simulink model "mech_motorcycle_stability"  (Simulink 6.0)
settings: Solver=ode45  StartTime=0.0  StopTime=3  RelTol=1e-3  AbsTol=1e-6
PreLoadFcn:
  | vu=53;mech_motorcycle_data
values from neighbouring files (symbols this model uses):
  Cf1 = -13.25+1.302*Zf-(1.39e-4)*Zf^2    [mech_motorcycle_data.m]
  Cf2 = 2.788+0.0165*Zf+(3.9e-6)*Zf^2    [mech_motorcycle_data.m]
  Cf3 = -0.06*Zf    [mech_motorcycle_data.m]
  Cfvf = -300+28.577*Zf-0.0143*Zf^2+(1.431e-6)*Zf^3+(3.347e-10)*Zf^4    [mech_motorcycle_data.m]
  Cfvr = -92.9+23.129*Zr-(4.663/1000)*Zr^2-(6.457e-7)*Zr^3+(1.887e-10)*Zr^4    [mech_motorcycle_data.m]
  Cmvf = -0.281+0.2442*Zf+(8.575e-5)*Zf^2    [mech_motorcycle_data.m]
  Cmvr = 9+0.3573*Zr + (3.378e-5)*Zr^2    [mech_motorcycle_data.m]
  Cr1 = 27.38+0.9727*Zr-(4e-6)*Zr^2    [mech_motorcycle_data.m]
  Cr2 = 2.056+0.01282*Zr+(4.928e-6)*Zr^2    [mech_motorcycle_data.m]
  Cr3 = -0.07*Zr    [mech_motorcycle_data.m]
  G = 9.81    [mech_motorcycle_data.m]
  m = 161    [mech_transmission_data.mat]
  Mfw = 26.5    [mech_motorcycle_data.m]    (also in mech_motorcycle_data_nonlinear.m = 25.6)
  Mp = 0.1    [mech_transmission_data.mat]
  Mrw = 26.5    [mech_motorcycle_data.m]    (also in mech_motorcycle_data_nonlinear.m = 25.6)
  N = 270    [mech_transmission_data.mat]
  Rf = 0.336    [mech_motorcycle_data.m]
  Rr = 0.321    [mech_motorcycle_data.m]
  sigmaf = 0.1012+(1.297e-4)*Zf-(3.267e-8)*Zf^2    [mech_motorcycle_data.m]
  sigmar = 0.03594+(1.941e-4)*Zr-(5.667e-8)*Zr^2+(5.728e-12)*Zr^3    [mech_motorcycle_data.m]
  Zf = ((Mf.value*(bb+kk)+Mr.value*bb+Mb.value*(bb-bb_b)+Mp.value*(bb-bb_p))*G-(vu^2)*(Dc.value*hh_cp+Lc.value*whl_bs/2))/whl_bs    [mech_motorcycle_data.m]
  Zr = (Mf.value+Mr.value+Mp.value+Mb.value)*G-Lc.value*vu^2-Zf    [mech_motorcycle_data.m]
undefined symbols (not defined in the file or in its folder): Crr1, Crr2, D_gamma, D_lamda, D_steer, D_v, D_zita, Dc, ifwy, Ifx, Ifxz, Ifz, Ipx, Ipxz, Ipz, irwx, irwy, Irx, Irxz, iry, Irz, k_gamma, k_lamda, k_steer, k_v, k_zita, Lc, Mb, Mf, Mr, rad, s
libraries: mblibv1 x43, simulink x8, aerospace x2
(part 1 of 2)
settings Model: Creator=gwood  LastModifiedBy=batserve  ExtModeAutoUpdateStatusClock=off
settings DataIOCC: SaveState=on  SignalLoggingName=logsOut  OutputTimes=0:0.5:20
settings OptimizationCC: BooleanDataType=off
settings DebuggingCC: CheckExecutionContextPreStartOutputMsg=on  CheckExecutionContextRuntimeOutputMsg=on  SolverPrmCheckMsg=none
settings HardwareCC: TargetUnknown=on

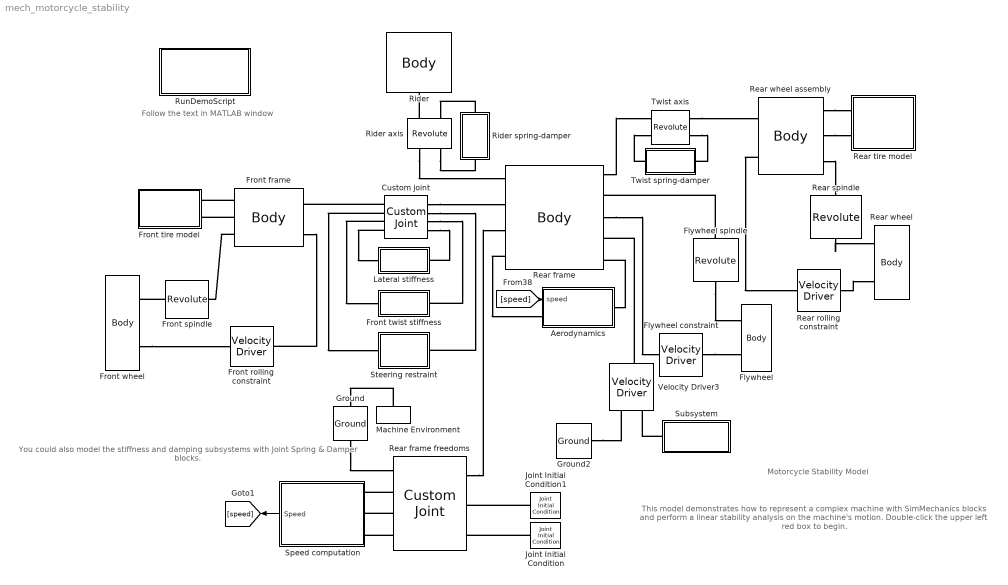
== system mech_motorcycle_stability ==
  note: Motorcycle Stability Model
  note: Follow the text in MATLAB window
  note: This model demonstrates how to represent
      | a complex machine with SimMechanics
      | blocks and perform a linear stability analysis
      | on the machine's motion. Double-click the
      | upper left red box to begin.
  note: You could also model the stiffness
      | and damping subsystems with
      | Joint Spring & Damper blocks.
  Aerodynamics : Subsystem
  Custom joint : mblibv1/Joints/Custom Joint  Orientation=left  PhysicalDomain=mechanical  SubClassName=custom_joint  LeftPortType=blob  RightPortType=blob  LConnTagsString=__newl0|SA1|SA2|SA3  RConnTagsString=__newr0|SA1|SA2|SA3  NumSAPorts=6  CutJoint=off  MarkAsCut=off  Primitives=prismatic_revolute_revolute  PrimitiveProps="P1$WORLD$[0 1 0]$prismatic#R1$WORLD$[cos(epsilon) 0  -sin(epsilon)]$revolute#R2$WORLD$[sin(epsilon) 0 cos(epsilon)]$revolute"  DialogClass=JointBlock
  Flywheel : mblibv1/Bodies/Body  PhysicalDomain=mechanical  SubClassName=Unknown  LeftPortType=workingframe  RightPortType=workingframe  LConnTagsString=CS2|CG  DialogClass=MechanicalBodyBlock  Mass=0  MassUnits=kg  InertiaUnits=kg*m^2  Inertia=[0 0 0;0 iry.value 0;0 0 0]  Shape=Cylinder  ShapeDims=[1 1]  ShapeUnits=m  ShapeUse=false  Density=1  DensityUnits=kg/m^3  DensityUse=false  CG=Left$CG$p1.coordinates$WORLD$WORLD$m$[0 0 0]$Euler X-Y-Z$deg$WORLD$true  WorkingFrames=Left$CS2$p1.coordinates$WORLD$WORLD$m$[0 0 0]$Euler X-Y-Z$deg$WORLD$true
  Flywheel constraint : mblibv1/Constraints &  Drivers/Velocity Driver  PhysicalDomain=mechanical  SubClassName=Unknown  LeftPortType=blob  RightPortType=blob  LConnTagsString=__newl0  RConnTagsString=__newr0  DialogClass=ConstantVelocityConstraint  NumSAPorts=0  Unit_V=m/s  Unit_Omega=rad/s  Coef_V_Base=[1 0 0]  Csys_V_Base=Base  Coef_Omega_Base=[0 0 0]  Csys_Omega_Base=Base  Coef_V_Follower=[0 0 0]  Csys_V_Follower=Follower  Coef_Omega_Follower=Rr*[0 -1 0]  Csys_Omega_Follower=Follower
  Flywheel spindle : mblibv1/Joints/Revolute  Orientation=down  PhysicalDomain=mechanical  SubClassName=Unknown  LeftPortType=blob  RightPortType=blob  LConnTagsString=__newl0  RConnTagsString=__newr0  NumSAPorts=0  CutJoint=off  MarkAsCut=off  Primitives=revolute  PrimitiveProps=R1$WORLD$[0 1 0]$revolute  DialogClass=JointBlock
  Front frame : mblibv1/Bodies/Body  Orientation=left  PhysicalDomain=mechanical  SubClassName=Unknown  LeftPortType=workingframe  RightPortType=workingframe  LConnTagsString=CS1|CS6  RConnTagsString=CS2|CS5|CS3  DialogClass=MechanicalBodyBlock  Mass=Mf.value  MassUnits=kg  InertiaUnits=kg*m^2  Inertia=[Ifx.value 0 Ifxz.value;0 0 0;Ifxz.value 0 Ifz.value]  Shape=Cylinder  ShapeDims=[1 1]  ShapeUnits=m  ShapeUse=false  Density=1  DensityUnits=kg/m^3  DensityUse=false  CG=Left$CG$p3.coordinates$WORLD$WORLD$m$[0 epsilon 0]$Euler X-Y-Z$rad$WORLD$false  WorkingFrames=Left$CS1$p8.coordinates$WORLD$WORLD$m$[0 0 0]$Euler X-Y-Z$deg$WORLD$true#Right$CS2$p11.coordinates$WORLD$WORLD$m$[0 0 0]$Euler X-Y-Z$deg$WORLD$true#Right$CS5$p11.coordinates$WORLD$WORLD$m$[0 0 0]$Euler X-Y-Z$deg$WORLD$true#Right$CS3$p6.coordinates$WORLD$WORLD$m$[0 0 0]$Euler X-Y-Z$deg$WORLD$true#Left$CS6$p6.coordinates$WORLD$WORLD$m$[0 0 0]$Euler X-Y-Z$deg$WORLD$true
  Front rolling constraint : mblibv1/Constraints &  Drivers/Velocity Driver  Orientation=left  PhysicalDomain=mechanical  SubClassName=Unknown  LeftPortType=blob  RightPortType=blob  LConnTagsString=__newl0  RConnTagsString=__newr0  DialogClass=ConstantVelocityConstraint  NumSAPorts=0  Unit_V=m/s  Unit_Omega=rad/s  Coef_V_Base=[1 0 0]  Csys_V_Base=Base  Coef_Omega_Base=[0 0 0]  Csys_Omega_Base=Base  Coef_V_Follower=[0 0 0]  Csys_V_Follower=Follower  Coef_Omega_Follower=Rf*[0 -1 0]  Csys_Omega_Follower=Follower
  Front spindle : mblibv1/Joints/Revolute  Orientation=left  PhysicalDomain=mechanical  SubClassName=Unknown  LeftPortType=blob  RightPortType=blob  LConnTagsString=__newl0  RConnTagsString=__newr0  NumSAPorts=0  CutJoint=off  MarkAsCut=off  Primitives=revolute  PrimitiveProps=R1$WORLD$[0 1 0]$revolute  DialogClass=JointBlock
  Front tire model : Subsystem  Orientation=left
  Front twist stiffness : Subsystem
  Front wheel : mblibv1/Bodies/Body  Orientation=left  PhysicalDomain=mechanical  SubClassName=Unknown  LeftPortType=workingframe  RightPortType=workingframe  LConnTagsString=CS1|CG  DialogClass=MechanicalBodyBlock  Mass=Mfw  MassUnits=kg  InertiaUnits=kg*m^2  Inertia=[0 0 0;0 ifwy.value 0;0 0 0]  Shape=Cylinder  ShapeDims=[1 1]  ShapeUnits=m  ShapeUse=false  Density=1  DensityUnits=kg/m^3  DensityUse=false  CG=Left$CG$p6.coordinates$WORLD$WORLD$m$[0 0 0]$Euler X-Y-Z$deg$WORLD$true  WorkingFrames=Left$CS1$p6.coordinates$WORLD$WORLD$m$[0 0 0]$Euler X-Y-Z$deg$WORLD$true
  Ground : mblibv1/Bodies/Ground  Orientation=down  Opaque=on  LeftPortType=env  RightPortType=workingframe  PhysicalDomain=Mechanical  DialogClass=GroundBlock  CoordPosition=p1.coordinates  CoordPositionUnits=m  StateVectorMgrId=-1  MachineId=[0 0]  ShowEnvPort=on
  Ground2 : mblibv1/Bodies/Ground  Opaque=on  LeftPortType=env  RightPortType=workingframe  PhysicalDomain=Mechanical  DialogClass=GroundBlock  CoordPosition=p7.coordinates  CoordPositionUnits=m  StateVectorMgrId=-1  MachineId=[0 0]  ShowEnvPort=off
  Joint Initial Condition : mblibv1/Sensors &  Actuators/Joint Initial Condition  Orientation=left  Opaque=on  PhysicalDomain=Mechanical  DialogClass=InitialConditionBlock  Primitive=R2  CoordPosition=0.005  Velocity=0.0  AngleUnits=rad  ArcVelocityUnits=rad/s  CoordPositionUnits=m  VelocityUnits=m/s  InitialConditions=P1$false$0$m$rad$0$m/s$rad/s#P2$false$0$m$rad$0$m/s$rad/s#P3$false$0$m$rad$0$m/s$rad/s#R1$false$0$m$rad$0$m/s$rad/s#R2$true$0.005$m$rad$0.0$m/s$rad/s#R3$false$0$m$rad$0$m/s$rad/s#S$false$0$m$rad$0$m/s$rad/s
  Joint Initial Condition1 : mblibv1/Sensors &  Actuators/Joint Initial Condition  Orientation=left  Opaque=on  PhysicalDomain=Mechanical  DialogClass=InitialConditionBlock  Primitive=R1  CoordPosition=0.0  Velocity=0.0  AngleUnits=rad  ArcVelocityUnits=rad/s  CoordPositionUnits=m  VelocityUnits=m/s  InitialConditions=P1$false$0$m$rad$0$m/s$rad/s#P2$false$0$m$rad$0$m/s$rad/s#P3$false$0$m$rad$0$m/s$rad/s#R1$true$0.0$m$rad$0.0$m/s$rad/s#R2$false$0$m$rad$0$m/s$rad/s#R3$false$0$m$rad$0$m/s$rad/s#S$false$0$m$rad$0$m/s$rad/s
  Lateral stiffness : Subsystem
  Machine Environment : mblibv1/Bodies/Machine Environment  Tag=Factory ground  Orientation=up  DialogController=MECH.DialogSource  Opaque=on  PortType=env  PhysicalDomain=Mechanical  DialogTemplateClass=MECH.MachineEnvironment  SyncWhenCopied=off  Gravity=[0;0;G]  GravityUnits=m/s^2  GravityAsSignal=off  Dimensionality=3D Only  AnalysisType=Forward dynamics  LinearAssemblyTolerance=1e-3  LinearAssemblyToleranceUnits=m  AngularAssemblyTolerance=1e-3  AngularAssemblyToleranceUnits=rad  ConstraintSolverType=Stabilizing  ConstraintRelTolerance=1e-4  ConstraintAbsTolerance=1e-4  UseRobustSingularityHandling=off  StatePerturbationType=Fixed  PerturbationSize=1e-5  VisualizeMachine=on
  Rear spindle : mblibv1/Joints/Revolute  Orientation=down  PhysicalDomain=mechanical  SubClassName=Unknown  LeftPortType=blob  RightPortType=blob  LConnTagsString=__newl0  RConnTagsString=__newr0  NumSAPorts=0  CutJoint=off  MarkAsCut=off  Primitives=revolute  PrimitiveProps=R1$WORLD$[0 1 0]$revolute  DialogClass=JointBlock
  Rear frame : mblibv1/Bodies/Body  PhysicalDomain=mechanical  SubClassName=Unknown  LeftPortType=workingframe  RightPortType=workingframe  LConnTagsString=CS1|CS3|CS6|CS9  RConnTagsString=CS2|CS7|CS8|CS11|CS10  DialogClass=MechanicalBodyBlock  Mass=Mr.value  MassUnits=kg  InertiaUnits=kg*m^2  Inertia=[Irx.value 0 Irxz.value;0 0 0;Irxz.value 0 Irz.value]  Shape=Cylinder  ShapeDims=[1 1]  ShapeUnits=m  ShapeUse=false  Density=1  DensityUnits=kg/m^3  DensityUse=false  CG=Right$CG$p1.coordinates$WORLD$WORLD$m$[0 0 0]$Euler X-Y-Z$deg$WORLD$false  WorkingFrames=Left$CS1$p9.coordinates$WORLD$WORLD$m$[0 0 0]$Euler X-Y-Z$deg$WORLD$true#Right$CS2$p7.coordinates$WORLD$WORLD$m$[0 0 0]$Euler X-Y-Z$deg$WORLD$true#Left$CS3$p8.coordinates$WORLD$WORLD$m$[0 0 0]$Euler X-Y-Z$deg$WORLD$true#Left$CS6$p1.coordinates$WORLD$WORLD$m$[0 0 0]$Euler X-Y-Z$deg$WORLD$true#Right$CS7$p1.coordinates$WORLD$WORLD$m$[0 0 0]$Euler X-Y-Z$deg$WORLD$true#Right$CS8$p1.coordinates$WORLD$WORLD$m$[0 0 0]$Euler X-Y-Z$deg$WORLD$true#Right$CS11$p10.coordinates$WORLD$WORLD$m$[0 0 0]$Euler X-Y-Z$deg$WORLD$true#Left$CS9$p12.coordinates$WORLD$WORLD$m$[0 0 0]$Euler X-Y-Z$deg$WORLD$true#Right$CS10$p12.coordinates$WORLD$WORLD$m$[0 0 0]$Euler X-Y-Z$deg$WORLD$true
  Rear frame freedoms : mblibv1/Joints/Custom Joint  PhysicalDomain=mechanical  SubClassName=custom_joint  LeftPortType=blob  RightPortType=blob  LConnTagsString=__newl0|SA1|SA2|SA3  RConnTagsString=__newr0|SA1|SA2  NumSAPorts=5  CutJoint=off  MarkAsCut=off  Primitives=prismatic_prismatic_revolute_revolute  PrimitiveProps=P1$WORLD$[1 0 0]$prismatic#P2$WORLD$[0 1 0]$prismatic#R1$WORLD$[0 0 1]$revolute#R2$WORLD$[1 0 0]$revolute  DialogClass=JointBlock
  Rear rolling constraint : mblibv1/Constraints &  Drivers/Velocity Driver  PhysicalDomain=mechanical  SubClassName=Unknown  LeftPortType=blob  RightPortType=blob  LConnTagsString=__newl0  RConnTagsString=__newr0  DialogClass=ConstantVelocityConstraint  NumSAPorts=0  Unit_V=m/s  Unit_Omega=rad/s  Coef_V_Base=[1 0 0]  Csys_V_Base=Base  Coef_Omega_Base=[0 0 0]  Csys_Omega_Base=Base  Coef_V_Follower=[0 0 0]  Csys_V_Follower=Follower  Coef_Omega_Follower=Rr*[0 -1 0]  Csys_Omega_Follower=Follower
  Rear tire model : Subsystem
  Rear wheel : mblibv1/Bodies/Body  PhysicalDomain=mechanical  SubClassName=Unknown  LeftPortType=workingframe  RightPortType=workingframe  LConnTagsString=CS1|CG  DialogClass=MechanicalBodyBlock  Mass=Mrw  MassUnits=kg  InertiaUnits=kg*m^2  Inertia=[irwx.value 0 0;0 irwy.value 0;0 0 irwx.value]  Shape=Cylinder  ShapeDims=[1 1]  ShapeUnits=m  ShapeUse=false  Density=1  DensityUnits=kg/m^3  DensityUse=false  CG=Left$CG$p5.coordinates$WORLD$WORLD$m$[0 0 0]$Euler X-Y-Z$deg$WORLD$true  WorkingFrames=Left$CS1$p5.coordinates$WORLD$WORLD$m$[0 0 0]$Euler X-Y-Z$deg$WORLD$true
  Rear wheel assembly : mblibv1/Bodies/Body  PhysicalDomain=mechanical  SubClassName=Unknown  LeftPortType=workingframe  RightPortType=workingframe  LConnTagsString=CS1|CS6  RConnTagsString=CS2|CS5|CS3  DialogClass=MechanicalBodyBlock  Mass=Mb.value  MassUnits=kg  InertiaUnits=kg*m^2  Inertia=zeros(3,3)  Shape=Cylinder  ShapeDims=[1 1]  ShapeUnits=m  ShapeUse=false  Density=1  DensityUnits=kg/m^3  DensityUse=false  CG=Left$CG$p2.coordinates$WORLD$WORLD$m$[0 0 0]$Euler X-Y-Z$deg$WORLD$false  WorkingFrames=Left$CS1$p7.coordinates$WORLD$WORLD$m$[0 0 0]$Euler X-Y-Z$deg$WORLD$true#Right$CS2$p10.coordinates$WORLD$WORLD$m$[0 0 0]$Euler X-Y-Z$deg$WORLD$true#Right$CS5$p10.coordinates$WORLD$WORLD$m$[0 0 0]$Euler X-Y-Z$deg$WORLD$true#Right$CS3$p5.coordinates$WORLD$WORLD$m$[0 0 0]$Euler X-Y-Z$deg$WORLD$true#Left$CS6$p5.coordinates$WORLD$WORLD$m$[0 0 0]$Euler X-Y-Z$deg$WORLD$true
  Rider : mblibv1/Bodies/Body  Orientation=up  PhysicalDomain=mechanical  SubClassName=Unknown  LeftPortType=workingframe  RightPortType=workingframe  LConnTagsString=CS1  DialogClass=MechanicalBodyBlock  Mass=Mp.value  MassUnits=kg  InertiaUnits=kg*m^2  Inertia=[Ipx.value 0 Ipxz.value;0 0 0;Ipxz.value 0 Ipz.value]  Shape=Cylinder  ShapeDims=[1 1]  ShapeUnits=m  ShapeUse=false  Density=1  DensityUnits=kg/m^3  DensityUse=false  CG=Left$CG$p4.coordinates$WORLD$WORLD$m$[0 0 0]$Euler X-Y-Z$deg$WORLD$false  WorkingFrames=Left$CS1$p9.coordinates$WORLD$WORLD$m$[0 0 0]$Euler X-Y-Z$deg$WORLD$true
  Rider axis : mblibv1/Joints/Revolute  Orientation=up  PhysicalDomain=mechanical  SubClassName=Unknown  LeftPortType=blob  RightPortType=blob  LConnTagsString=__newl0|SA1  RConnTagsString=__newr0|SA1  NumSAPorts=2  CutJoint=off  MarkAsCut=off  Primitives=revolute  PrimitiveProps=R1$WORLD$[1 0 0]$revolute  DialogClass=JointBlock
  Rider spring-damper : Subsystem  Orientation=down
  RunDemoScript : Subsystem
      settings: OpenFcn=mech_motorcycle_stability_demo
      mask Display: disp('Double-click\nhere to\nstart Demo')
  Speed computation : Subsystem  Orientation=left
  Steering restraint : Subsystem
  Subsystem : Subsystem  Orientation=left
  Twist axis : mblibv1/Joints/Revolute  PhysicalDomain=mechanical  SubClassName=Unknown  LeftPortType=blob  RightPortType=blob  LConnTagsString=__newl0|SA1  RConnTagsString=__newr0|SA1  NumSAPorts=2  CutJoint=off  MarkAsCut=off  Primitives=revolute  PrimitiveProps=R1$WORLD$[sin(epsilon1) 0 cos(epsilon1)]$revolute  DialogClass=JointBlock
  Twist spring-damper : Subsystem
  Velocity Driver3 : mblibv1/Constraints &  Drivers/Velocity Driver  Orientation=up  PhysicalDomain=mechanical  SubClassName=Unknown  LeftPortType=blob  RightPortType=blob  LConnTagsString=__newl0|SA1  RConnTagsString=__newr0  DialogClass=ConstantVelocityConstraint  NumSAPorts=1  Unit_V=m/s  Unit_Omega=rad/s  Coef_V_Base=[1 0 0]  Csys_V_Base=Base  Coef_Omega_Base=[0 0 0]  Csys_Omega_Base=Base  Coef_V_Follower=[1 0 0]  Csys_V_Follower=Follower  Coef_Omega_Follower=[0 0 0]  Csys_Omega_Follower=Follower
  wires:
  [speed] -> Aerodynamics/1(speed)
  Speed computation/1(Speed) -> [speed]
  connections:
  Rider axis/LConn1 -- Rear frame/LConn1
  Custom joint/LConn1 -- Rear frame/LConn2
  Front frame/RConn3 -- Front spindle/LConn1
  Custom joint/RConn1 -- Front frame/LConn1
  Rider axis/LConn2 -- Rider spring-damper/RConn1
  Rider axis/RConn1 -- Rider/LConn1
  Rider spring-damper/LConn1 -- Rider axis/RConn2
  Custom joint/LConn4 -- Lateral stiffness/RConn1
  Custom joint/RConn4 -- Lateral stiffness/LConn1
  Custom joint/RConn3 -- Front twist stiffness/LConn1
  Custom joint/LConn3 -- Front twist stiffness/RConn1
  Custom joint/LConn2 -- Steering restraint/RConn1
  Custom joint/RConn2 -- Steering restraint/LConn1
  Front frame/RConn1 -- Front tire model/LConn1
  Front frame/RConn2 -- Front tire model/LConn2
  Rear wheel assembly/RConn3 -- Rear spindle/LConn1
  Twist axis/RConn1 -- Rear wheel assembly/LConn1
  Rear frame/LConn4 -- Aerodynamics/LConn1
  Front frame/LConn2 -- Front rolling constraint/LConn1
  Rear wheel assembly/LConn2 -- Rear rolling constraint/LConn1
  Flywheel spindle/LConn1 -- Rear frame/RConn2
  Rear frame/RConn3 -- Flywheel constraint/LConn1
  Velocity Driver3/RConn1 -- Rear frame/RConn4
  Front spindle/RConn1 -- Front wheel/LConn1
  Front wheel/LConn2 -- Front rolling constraint/RConn1
  Rear frame freedoms/RConn1 -- Rear frame/LConn3
  Ground/RConn1 -- Rear frame freedoms/LConn1
  Rear frame freedoms/LConn2 -- Speed computation/LConn1
  Rear frame freedoms/LConn3 -- Speed computation/LConn2
  Rear frame freedoms/LConn4 -- Speed computation/LConn3
  Joint Initial Condition/RConn1 -- Rear frame freedoms/RConn3
  Joint Initial Condition1/RConn1 -- Rear frame freedoms/RConn2
  Aerodynamics/RConn1 -- Rear frame/RConn5
  Twist axis/RConn2 -- Twist spring-damper/RConn1
  Rear wheel assembly/RConn1 -- Rear tire model/LConn1
  Rear wheel assembly/RConn2 -- Rear tire model/LConn2
  Ground2/RConn1 -- Velocity Driver3/LConn1
  Subsystem/RConn1 -- Velocity Driver3/LConn2
  Rear spindle/RConn1 -- Rear wheel/LConn1
  Rear rolling constraint/RConn1 -- Rear wheel/LConn2
  Flywheel spindle/RConn1 -- Flywheel/LConn1
  Flywheel constraint/RConn1 -- Flywheel/LConn2
  Rear frame/RConn1 -- Twist axis/LConn1
  Twist spring-damper/LConn1 -- Twist axis/LConn2
  Machine Environment/RConn1 -- Ground/LConn1

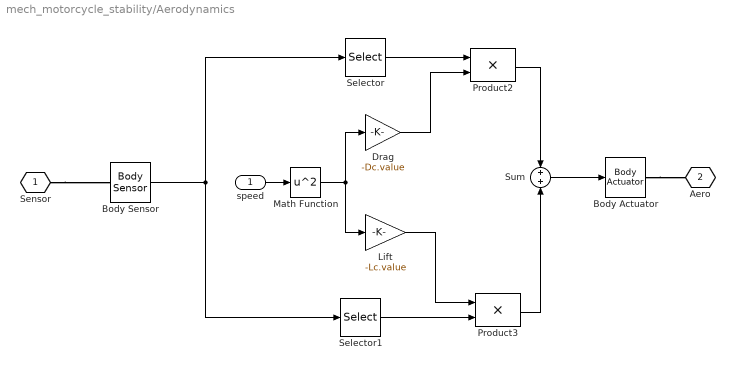
== system mech_motorcycle_stability/Aerodynamics ==
  speed : Inport  Port=1  LatchInput=off
  Body Actuator : mblibv1/Sensors &  Actuators/Body Actuator  Opaque=on  PhysicalDomain=Mechanical  PortType=blob  ActuationStyle=Force  AngleUnits=deg  ArcVelocityUnits=deg/s  ArcAccelerationUnits=deg/s^2  CoordPositionUnits=m  VelocityUnits=m/s  AccelerationUnits=m/s^2  ForceUnits=N  TorqueUnits=N-m  ActiveIO=on  Width=3  DialogClass=MechanicalActuatorBlock  ReferenceFrame=Absolute (World)  Angle=off  CoordPosition=on  Force=on  Torque=off
  Body Sensor : mblibv1/Sensors &  Actuators/Body Sensor  Opaque=on  PhysicalDomain=Mechanical  PortType=blob  Muxed=on  Pose=on  Angle=on  AngleUnits=deg  ArcVelocity=off  ArcVelocityUnits=deg/s  ArcAcceleration=off  ArcAccelerationUnits=deg/s^2  CoordPosition=off  CoordPositionUnits=m  Velocity=off  VelocityUnits=m/s  Acceleration=off  AccelerationUnits=m/s^2  Quaternion=on  QuaternionDT=off  QuaternionDDT=off  QuaternionUnits=off  OutputVector=[ 9 ]  ActiveIO=on  Width=9  DialogClass=MechanicalSensorBlock  ReferenceFrame=Absolute (World)
  Drag : Gain  Gain=-Dc.value  SaturateOnIntegerOverflow=on
  Lift : Gain  Gain=-Lc.value  SaturateOnIntegerOverflow=on
  Math Function : Math  Operator=square  SaturateOnIntegerOverflow=on
  Product2 : Product  SaturateOnIntegerOverflow=on  InputSameDT=on
  Product3 : Product  SaturateOnIntegerOverflow=on  InputSameDT=on
  Selector : Selector  Elements=[1:3]  InputPortWidth=9
  Selector1 : Selector  Elements=[7:9]  InputPortWidth=9
  Sum : Sum  SaturateOnIntegerOverflow=on  InputSameDT=on
  Sensor : PMIOPort  Port=1  Side=Left
  Aero : PMIOPort  Orientation=left  Port=2  Side=Right
  wires:
  speed/1 -> Math Function/1
  Math Function/1 -> Drag/1, Lift/1
  Lift/1 -> Product3/1
  Selector/1 -> Product2/1
  Body Sensor/1 -> Selector/1, Selector1/1
  Sum/1 -> Body Actuator/1
  Product2/1 -> Sum/1
  Product3/1 -> Sum/2
  Drag/1 -> Product2/2
  Selector1/1 -> Product3/2
  connections:
  Body Actuator/RConn1 -- Aero/RConn1
  Sensor/RConn1 -- Body Sensor/LConn1

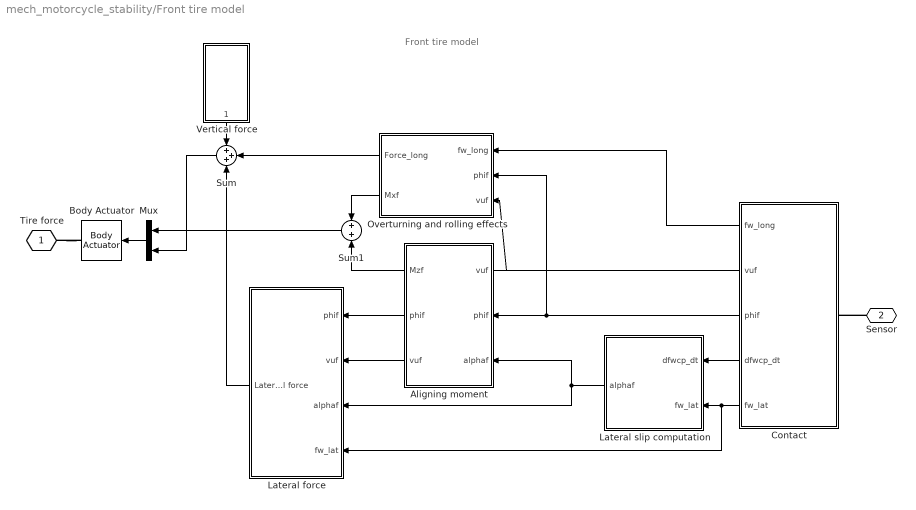
== system mech_motorcycle_stability/Front tire model ==
  note: Front tire model
  Aligning moment : Subsystem  Orientation=left
  Body Actuator : mblibv1/Sensors &  Actuators/Body Actuator  Orientation=left  Opaque=on  PhysicalDomain=Mechanical  PortType=blob  ActuationStyle=Force  AngleUnits=deg  ArcVelocityUnits=deg/s  ArcAccelerationUnits=deg/s^2  CoordPositionUnits=m  VelocityUnits=m/s  AccelerationUnits=m/s^2  ForceUnits=N  TorqueUnits=N-m  ActiveIO=on  Width=6  DialogClass=MechanicalActuatorBlock  ReferenceFrame=Absolute (World)  Angle=off  CoordPosition=off  Force=on  Torque=on
  Contact : Subsystem  Orientation=left
  Lateral force : Subsystem  Orientation=left
  Lateral slip computation : Subsystem  Orientation=left
  Mux : Mux  Orientation=left  Inputs=2
  Overturning and rolling effects : Subsystem  Orientation=left
  Sum : Sum  Orientation=left  Inputs=+++  SaturateOnIntegerOverflow=on  InputSameDT=on
  Sum1 : Sum  Orientation=left  SaturateOnIntegerOverflow=on  InputSameDT=on
  Vertical force : Subsystem  Orientation=down
  Tire force : PMIOPort  Tag=PMCPort  Port=1  Side=Left
  Sensor : PMIOPort  Orientation=left  Port=2  Side=Left
  wires:
  Vertical force/1(Force_vert) -> Sum/1
  Aligning moment/3("vuf ") -> Lateral force/2(vuf)
  Aligning moment/2("phif ") -> Lateral force/1(phif)
  Aligning moment/1(Mzf) -> Sum1/2
  Overturning and rolling effects/2(Mxf) -> Sum1/1
  Lateral force/1(Lateral force) -> Sum/3
  Overturning and rolling effects/1(Force_long) -> Sum/2
  Contact/4(dfwcp_dt) -> Lateral slip computation/1(dfwcp_dt)
  Contact/5(fw_lat) -> Lateral slip computation/2(fw_lat), Lateral force/4(fw_lat)
  Contact/3(phif) -> Aligning moment/2(phif), Overturning and rolling effects/2(phif)
  Contact/1(fw_long) -> Overturning and rolling effects/1(fw_long)
  Contact/2(vuf) -> Aligning moment/1(vuf), Overturning and rolling effects/3(vuf)
  Lateral slip computation/1(alphaf) -> Aligning moment/3(alphaf), Lateral force/3(alphaf)
  Sum1/1 -> Mux/1
  Sum/1 -> Mux/2
  Mux/1 -> Body Actuator/1
  connections:
  Body Actuator/RConn1 -- Tire force/RConn1
  Sensor/RConn1 -- Contact/LConn1

== system mech_motorcycle_stability/Front twist stiffness ==
  note: Twist stiffness model for bending flexibility
  note: Press any key to continue
  Damping : Gain  Gain=-D_gamma.value  SaturateOnIntegerOverflow=on
  Demux : Demux  Outputs=2
  Initial Force : Constant  Value=0
  Joint Actuator : mblibv1/Sensors &  Actuators/Joint Actuator  Opaque=on  PhysicalDomain=Mechanical  PortType=blob  ActuationStyle=Force  AngleUnits=rad  ArcVelocityUnits=rad/s  ArcAccelerationUnits=rad/s^2  CoordPositionUnits=m  VelocityUnits=m/s  AccelerationUnits=m/s^2  ForceUnits=N  TorqueUnits=N-m  ActiveIO=on  Width=1  DialogClass=MechanicalActuatorBlock  Primitive=R1  ReferenceFrame=Absolute (INERTIAL)
  Joint Sensor : mblibv1/Sensors &  Actuators/Joint Sensor  Opaque=on  PhysicalDomain=Mechanical  PortType=blob  Muxed=on  Pose=off  Angle=on  AngleUnits=rad  ArcVelocity=on  ArcVelocityUnits=rad/s  ArcAcceleration=off  ArcAccelerationUnits=deg/s^2  CoordPosition=on  CoordPositionUnits=m  Velocity=on  VelocityUnits=m/s  Acceleration=off  AccelerationUnits=m/s^2  Quaternion=on  QuaternionDT=off  QuaternionDDT=off  QuaternionUnits=off  OutputVector=[ 1 1 ]  ActiveIO=on  Width=2  DialogClass=MechanicalSensorBlock  Primitive=R1  Force=off  ForceUnits=N  Torque=off  TorqueUnits=N-m  ReferenceFrame=Absolute (INERTIAL)  ReactionSensedSide=Base  ReactionReferenceFrame=Absolute (World)  ReactionForce=off  ReactionForceUnits=N  ReactionMoment=off  ReactionMomentUnits=N-m
  Stiffness : Gain  Gain=-k_gamma.value  SaturateOnIntegerOverflow=on
  Sum : Sum  Inputs=+++  SaturateOnIntegerOverflow=on  InputSameDT=on
  S : PMIOPort  Port=1  Side=Left
  A : PMIOPort  Orientation=left  Port=2  Side=Right
  wires:
  Joint Sensor/1 -> Demux/1
  Demux/1 -> Stiffness/1  "Rotation (rad)"
  Demux/2 -> Damping/1  "Rotation rate (rad/s)"
  Damping/1 -> Sum/2
  Stiffness/1 -> Sum/1
  Initial Force/1 -> Sum/3
  Sum/1 -> Joint Actuator/1  "Torque (Nm)"
  connections:
  S/RConn1 -- Joint Sensor/LConn1
  Joint Actuator/RConn1 -- A/RConn1

== system mech_motorcycle_stability/Lateral stiffness ==
  note: Lateral stiffness model for transverse flexibility
  note: Press any key to continue
  Damping : Gain  Gain=-D_v.value  SaturateOnIntegerOverflow=on
  Demux : Demux  Outputs=2
  Initial Force : Constant  Value=0
  Joint Actuator : mblibv1/Sensors &  Actuators/Joint Actuator  Opaque=on  PhysicalDomain=Mechanical  PortType=blob  ActuationStyle=Force  AngleUnits=rad  ArcVelocityUnits=rad/s  ArcAccelerationUnits=rad/s^2  CoordPositionUnits=m  VelocityUnits=m/s  AccelerationUnits=m/s^2  ForceUnits=N  TorqueUnits=N-m  ActiveIO=on  Width=1  DialogClass=MechanicalActuatorBlock  Primitive=P1  ReferenceFrame=Absolute (INERTIAL)
  Joint Sensor : mblibv1/Sensors &  Actuators/Joint Sensor  Opaque=on  PhysicalDomain=Mechanical  PortType=blob  Muxed=on  Pose=off  Angle=on  AngleUnits=rad  ArcVelocity=on  ArcVelocityUnits=rad/s  ArcAcceleration=off  ArcAccelerationUnits=deg/s^2  CoordPosition=on  CoordPositionUnits=m  Velocity=on  VelocityUnits=m/s  Acceleration=off  AccelerationUnits=m/s^2  Quaternion=on  QuaternionDT=off  QuaternionDDT=off  QuaternionUnits=off  OutputVector=[ 1 1 ]  ActiveIO=on  Width=2  DialogClass=MechanicalSensorBlock  Primitive=P1  Force=off  ForceUnits=N  Torque=off  TorqueUnits=N-m  ReferenceFrame=Absolute (INERTIAL)  ReactionSensedSide=Base  ReactionReferenceFrame=Absolute (World)  ReactionForce=off  ReactionForceUnits=N  ReactionMoment=off  ReactionMomentUnits=N-m
  Stiffness : Gain  Gain=-k_v.value  SaturateOnIntegerOverflow=on
  Sum : Sum  Inputs=+++  SaturateOnIntegerOverflow=on  InputSameDT=on
  S : PMIOPort  Port=1  Side=Left
  A : PMIOPort  Orientation=left  Port=2  Side=Right
  wires:
  Initial Force/1 -> Sum/3
  Stiffness/1 -> Sum/1
  Damping/1 -> Sum/2
  Demux/2 -> Damping/1  "Velocity (m/s)"
  Demux/1 -> Stiffness/1  "Displacement (m)"
  Joint Sensor/1 -> Demux/1
  Sum/1 -> Joint Actuator/1  "Lateral force (N)"
  connections:
  Joint Actuator/RConn1 -- A/RConn1
  S/RConn1 -- Joint Sensor/LConn1

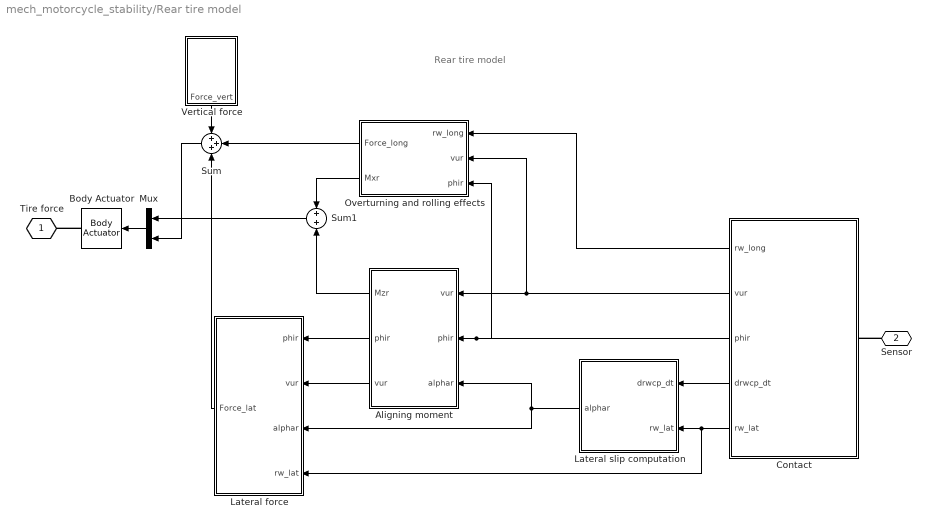
== system mech_motorcycle_stability/Rear tire model ==
  note: Rear tire model
  Aligning moment : Subsystem  Orientation=left
  Body Actuator : mblibv1/Sensors &  Actuators/Body Actuator  Orientation=left  Opaque=on  PhysicalDomain=Mechanical  PortType=blob  ActuationStyle=Force  AngleUnits=deg  ArcVelocityUnits=deg/s  ArcAccelerationUnits=deg/s^2  CoordPositionUnits=m  VelocityUnits=m/s  AccelerationUnits=m/s^2  ForceUnits=N  TorqueUnits=N-m  ActiveIO=on  Width=6  DialogClass=MechanicalActuatorBlock  ReferenceFrame=Absolute (World)  Angle=off  CoordPosition=off  Force=on  Torque=on
  Contact : Subsystem  Orientation=left
  Lateral force : Subsystem  Orientation=left
  Lateral slip computation : Subsystem  Orientation=left
  Mux : Mux  Orientation=left  Inputs=2
  Overturning and rolling effects : Subsystem  Orientation=left
  Sum : Sum  Orientation=left  Inputs=+++  SaturateOnIntegerOverflow=on  InputSameDT=on
  Sum1 : Sum  Orientation=left  SaturateOnIntegerOverflow=on  InputSameDT=on
  Vertical force : Subsystem  Orientation=down
  Tire force : PMIOPort  Tag=PMCPort  Port=1  Side=Left
  Sensor : PMIOPort  Orientation=left  Port=2  Side=Left
  wires:
  Aligning moment/2("phir ") -> Lateral force/1(phir)
  Aligning moment/3("vur ") -> Lateral force/2(vur)
  Aligning moment/1(Mzr) -> Sum1/2
  Overturning and rolling effects/2(Mxr) -> Sum1/1
  Lateral force/1(Force_lat) -> Sum/3
  Overturning and rolling effects/1(Force_long) -> Sum/2
  Contact/4(drwcp_dt) -> Lateral slip computation/1(drwcp_dt)
  Contact/5(rw_lat) -> Lateral slip computation/2(rw_lat), Lateral force/4(rw_lat)
  Contact/3(phir) -> Aligning moment/2(phir), Overturning and rolling effects/3(phir)
  Contact/2(vur) -> Aligning moment/1(vur), Overturning and rolling effects/2(vur)
  Contact/1(rw_long) -> Overturning and rolling effects/1(rw_long)
  Sum1/1 -> Mux/1
  Sum/1 -> Mux/2
  Mux/1 -> Body Actuator/1
  Vertical force/1(Force_vert) -> Sum/1
  Lateral slip computation/1(alphar) -> Aligning moment/3(alphar), Lateral force/3(alphar)
  connections:
  Sensor/RConn1 -- Contact/LConn1
  Body Actuator/RConn1 -- Tire force/RConn1

== system mech_motorcycle_stability/Rider spring-damper ==
  note: Rider stiffness and damping model
  note: Press any key to continue
  Damping : Gain  Gain=-D_zita.value  SaturateOnIntegerOverflow=on
  Demux : Demux  Outputs=2
  Initial Force : Constant  Value=0
  Joint Actuator : mblibv1/Sensors &  Actuators/Joint Actuator  Opaque=on  PhysicalDomain=Mechanical  PortType=blob  ActuationStyle=Force  AngleUnits=deg  ArcVelocityUnits=deg/s  ArcAccelerationUnits=deg/s^2  CoordPositionUnits=m  VelocityUnits=m/s  AccelerationUnits=m/s^2  ForceUnits=N  TorqueUnits=N-m  ActiveIO=on  Width=1  DialogClass=MechanicalActuatorBlock  Primitive=R1  ReferenceFrame=Absolute (INERTIAL)
  Joint Sensor : mblibv1/Sensors &  Actuators/Joint Sensor  Opaque=on  PhysicalDomain=Mechanical  PortType=blob  Muxed=on  Pose=off  Angle=on  AngleUnits=rad  ArcVelocity=on  ArcVelocityUnits=rad/s  ArcAcceleration=off  ArcAccelerationUnits=deg/s^2  CoordPosition=on  CoordPositionUnits=m  Velocity=on  VelocityUnits=m/s  Acceleration=off  AccelerationUnits=m/s^2  Quaternion=on  QuaternionDT=off  QuaternionDDT=off  QuaternionUnits=off  OutputVector=[ 1 1 ]  ActiveIO=on  Width=2  DialogClass=MechanicalSensorBlock  Primitive=R1  Force=off  ForceUnits=N  Torque=off  TorqueUnits=N-m  ReferenceFrame=Absolute (INERTIAL)  ReactionSensedSide=Base  ReactionReferenceFrame=Absolute (World)  ReactionForce=off  ReactionForceUnits=N  ReactionMoment=off  ReactionMomentUnits=N-m
  Stiffness : Gain  Gain=-k_zita.value  SaturateOnIntegerOverflow=on
  Sum : Sum  Inputs=+++  SaturateOnIntegerOverflow=on  InputSameDT=on
  S : PMIOPort  Port=1  Side=Left
  A : PMIOPort  Orientation=left  Port=2  Side=Right
  wires:
  Sum/1 -> Joint Actuator/1  "Torque (Nm)"
  Initial Force/1 -> Sum/3
  Stiffness/1 -> Sum/1
  Damping/1 -> Sum/2
  Demux/2 -> Damping/1  "Angular velocity (rad/s)"
  Demux/1 -> Stiffness/1  "Angle (rad)"
  Joint Sensor/1 -> Demux/1
  connections:
  Joint Actuator/RConn1 -- A/RConn1
  S/RConn1 -- Joint Sensor/LConn1

== system mech_motorcycle_stability/RunDemoScript ==

== system mech_motorcycle_stability/Speed computation ==
  Joint Sensor : mblibv1/Sensors &  Actuators/Joint Sensor  Orientation=left  Opaque=on  PhysicalDomain=Mechanical  PortType=blob  Muxed=on  Pose=off  Angle=on  AngleUnits=deg  ArcVelocity=off  ArcVelocityUnits=deg/s  ArcAcceleration=off  ArcAccelerationUnits=deg/s^2  CoordPosition=off  CoordPositionUnits=m  Velocity=on  VelocityUnits=m/s  Acceleration=off  AccelerationUnits=m/s^2  Quaternion=on  QuaternionDT=off  QuaternionDDT=off  QuaternionUnits=off  OutputVector=[ 1 ]  ActiveIO=on  Width=1  DialogClass=MechanicalSensorBlock  Primitive=P1  Force=off  ForceUnits=N  Torque=off  TorqueUnits=N-m  ReferenceFrame=Absolute (INERTIAL)  ReactionSensedSide=Base  ReactionReferenceFrame=Absolute (World)  ReactionForce=off  ReactionForceUnits=N  ReactionMoment=off  ReactionMomentUnits=N-m
  Joint Sensor1 : mblibv1/Sensors &  Actuators/Joint Sensor  Orientation=left  Opaque=on  PhysicalDomain=Mechanical  PortType=blob  Muxed=on  Pose=off  Angle=on  AngleUnits=deg  ArcVelocity=off  ArcVelocityUnits=deg/s  ArcAcceleration=off  ArcAccelerationUnits=deg/s^2  CoordPosition=off  CoordPositionUnits=m  Velocity=on  VelocityUnits=m/s  Acceleration=off  AccelerationUnits=m/s^2  Quaternion=on  QuaternionDT=off  QuaternionDDT=off  QuaternionUnits=off  OutputVector=[ 1 ]  ActiveIO=on  Width=1  DialogClass=MechanicalSensorBlock  Primitive=P2  Force=off  ForceUnits=N  Torque=off  TorqueUnits=N-m  ReferenceFrame=Absolute (INERTIAL)  ReactionSensedSide=Base  ReactionReferenceFrame=Absolute (World)  ReactionForce=off  ReactionForceUnits=N  ReactionMoment=off  ReactionMomentUnits=N-m
  Joint Sensor2 : mblibv1/Sensors &  Actuators/Joint Sensor  Orientation=left  Opaque=on  PhysicalDomain=Mechanical  PortType=blob  Muxed=on  Pose=off  Angle=on  AngleUnits=rad  ArcVelocity=off  ArcVelocityUnits=rad/s  ArcAcceleration=off  ArcAccelerationUnits=deg/s^2  CoordPosition=off  CoordPositionUnits=m  Velocity=on  VelocityUnits=m/s  Acceleration=off  AccelerationUnits=m/s^2  Quaternion=on  QuaternionDT=off  QuaternionDDT=off  QuaternionUnits=off  OutputVector=[ 1 ]  ActiveIO=on  Width=1  DialogClass=MechanicalSensorBlock  Primitive=R1  Force=off  ForceUnits=N  Torque=off  TorqueUnits=N-m  ReferenceFrame=Absolute (INERTIAL)  ReactionSensedSide=Base  ReactionReferenceFrame=Absolute (World)  ReactionForce=off  ReactionForceUnits=N  ReactionMoment=off  ReactionMomentUnits=N-m
  Product : Product  Orientation=left  SaturateOnIntegerOverflow=on  InputSameDT=on
  Product1 : Product  Orientation=left  SaturateOnIntegerOverflow=on  InputSameDT=on
  Sum : Sum  Orientation=left  Inputs=|++  SaturateOnIntegerOverflow=on  InputSameDT=on
  Trigonometric Function : Trigonometry  Orientation=left  Operator=cos
  Trigonometric Function1 : Trigonometry  Orientation=left
  Sensor1 : PMIOPort  Orientation=left  Port=1  Side=Left
  Sensor2 : PMIOPort  Orientation=left  Port=2  Side=Left
  Sensor3 : PMIOPort  Orientation=left  Port=3  Side=Left
  Speed : Outport  Orientation=left
  wires:
  Joint Sensor/1 -> Product/1
  Joint Sensor1/1 -> Product1/1
  Trigonometric Function/1 -> Product/2
  Trigonometric Function1/1 -> Product1/2
  Product/1 -> Sum/1
  Product1/1 -> Sum/2
  Joint Sensor2/1 -> Trigonometric Function/1, Trigonometric Function1/1
  Sum/1 -> Speed/1
  connections:
  Sensor1/RConn1 -- Joint Sensor/LConn1
  Sensor2/RConn1 -- Joint Sensor1/LConn1
  Sensor3/RConn1 -- Joint Sensor2/LConn1

== system mech_motorcycle_stability/Steering restraint ==
  note: Steering restraint model for rider's arms
  note: Press any key to continue
  Damping : Gain  Gain=-D_steer.value  SaturateOnIntegerOverflow=on
  Demux : Demux  Outputs=2
  Joint Actuator : mblibv1/Sensors &  Actuators/Joint Actuator  Opaque=on  PhysicalDomain=Mechanical  PortType=blob  ActuationStyle=Force  AngleUnits=rad  ArcVelocityUnits=rad/s  ArcAccelerationUnits=rad/s^2  CoordPositionUnits=m  VelocityUnits=m/s  AccelerationUnits=m/s^2  ForceUnits=N  TorqueUnits=N-m  ActiveIO=on  Width=1  DialogClass=MechanicalActuatorBlock  Primitive=R2  ReferenceFrame=Absolute (INERTIAL)
  Joint Sensor : mblibv1/Sensors &  Actuators/Joint Sensor  Opaque=on  PhysicalDomain=Mechanical  PortType=blob  Muxed=on  Pose=off  Angle=on  AngleUnits=rad  ArcVelocity=on  ArcVelocityUnits=rad/s  ArcAcceleration=off  ArcAccelerationUnits=deg/s^2  CoordPosition=on  CoordPositionUnits=m  Velocity=on  VelocityUnits=m/s  Acceleration=off  AccelerationUnits=m/s^2  Quaternion=on  QuaternionDT=off  QuaternionDDT=off  QuaternionUnits=off  OutputVector=[ 1 1 ]  ActiveIO=on  Width=2  DialogClass=MechanicalSensorBlock  Primitive=R2  Force=off  ForceUnits=N  Torque=off  TorqueUnits=N-m  ReferenceFrame=Absolute (INERTIAL)  ReactionSensedSide=Base  ReactionReferenceFrame=Absolute (World)  ReactionForce=off  ReactionForceUnits=N  ReactionMoment=off  ReactionMomentUnits=N-m
  Scope : Scope
      settings: YMin=-0.00055  YMax=0.0005
  Stiffness : Gain  Gain=-k_steer.value  SaturateOnIntegerOverflow=on
  Sum : Sum  SaturateOnIntegerOverflow=on  InputSameDT=on
  S : PMIOPort  Port=1  Side=Left
  A : PMIOPort  Orientation=left  Port=2  Side=Right
  wires:
  Demux/2 -> Damping/1, Scope/1  "Angular velocity (rad/s)"
  Demux/1 -> Stiffness/1  "Angle (rad)"
  Joint Sensor/1 -> Demux/1
  Sum/1 -> Joint Actuator/1  "Torque (Nm)"
  Stiffness/1 -> Sum/1
  Damping/1 -> Sum/2
  connections:
  Joint Actuator/RConn1 -- A/RConn1
  S/RConn1 -- Joint Sensor/LConn1

== system mech_motorcycle_stability/Subsystem ==
  Constant : Constant  Value=-vu
  Constant1 : Constant  Orientation=left  Value=0
  Driver Actuator : mblibv1/Sensors &  Actuators/Driver Actuator  Orientation=up  Opaque=on  PhysicalDomain=Mechanical  DialogClass=ConstraintActuatorBlock  PortType=blob  AngleUnits=deg  ArcVelocityUnits=deg/s  ArcAccelerationUnits=deg/s^2  CoordPositionUnits=m  VelocityUnits=m/s  AccelerationUnits=m/s^2  ActiveIO=on  Width=2
  Mux : Mux  Orientation=up  Inputs=2
  DriverActuator : PMIOPort  Orientation=down  Port=1  Side=Right
  wires:
  Mux/1 -> Driver Actuator/1
  Constant/1 -> Mux/1
  Constant1/1 -> Mux/2
  connections:
  DriverActuator/RConn1 -- Driver Actuator/RConn1

== system mech_motorcycle_stability/Twist spring-damper ==
  note: Twist spring damper model
  note: Press any key to continue
  Damping : Gain  Gain=-D_lamda.value  SaturateOnIntegerOverflow=on
  Demux : Demux  Outputs=2
  Initial Force : Constant  Value=0
  Joint Actuator : mblibv1/Sensors &  Actuators/Joint Actuator  Opaque=on  PhysicalDomain=Mechanical  PortType=blob  ActuationStyle=Force  AngleUnits=rad  ArcVelocityUnits=rad/s  ArcAccelerationUnits=rad/s^2  CoordPositionUnits=m  VelocityUnits=m/s  AccelerationUnits=m/s^2  ForceUnits=N  TorqueUnits=N-m  ActiveIO=on  Width=1  DialogClass=MechanicalActuatorBlock  Primitive=R1  ReferenceFrame=Absolute (INERTIAL)
  Joint Sensor : mblibv1/Sensors &  Actuators/Joint Sensor  Opaque=on  PhysicalDomain=Mechanical  PortType=blob  Muxed=on  Pose=off  Angle=on  AngleUnits=rad  ArcVelocity=on  ArcVelocityUnits=rad/s  ArcAcceleration=off  ArcAccelerationUnits=deg/s^2  CoordPosition=on  CoordPositionUnits=m  Velocity=on  VelocityUnits=m/s  Acceleration=off  AccelerationUnits=m/s^2  Quaternion=on  QuaternionDT=off  QuaternionDDT=off  QuaternionUnits=off  OutputVector=[ 1 1 ]  ActiveIO=on  Width=2  DialogClass=MechanicalSensorBlock  Primitive=R1  Force=off  ForceUnits=N  Torque=off  TorqueUnits=N-m  ReferenceFrame=Absolute (INERTIAL)  ReactionSensedSide=Base  ReactionReferenceFrame=Absolute (World)  ReactionForce=off  ReactionForceUnits=N  ReactionMoment=off  ReactionMomentUnits=N-m
  Stiffness : Gain  Gain=-k_lamda.value  SaturateOnIntegerOverflow=on
  Sum : Sum  Inputs=+++  SaturateOnIntegerOverflow=on  InputSameDT=on
  S : PMIOPort  Port=1  Side=Left
  A : PMIOPort  Orientation=left  Port=2  Side=Right
  wires:
  Sum/1 -> Joint Actuator/1  "Torque (Nm)"
  Joint Sensor/1 -> Demux/1
  Demux/1 -> Stiffness/1  "Angle (rad)"
  Demux/2 -> Damping/1  "Angular velocity (rad/s)"
  Damping/1 -> Sum/2
  Stiffness/1 -> Sum/1
  Initial Force/1 -> Sum/3
  connections:
  S/RConn1 -- Joint Sensor/LConn1
  Joint Actuator/RConn1 -- A/RConn1

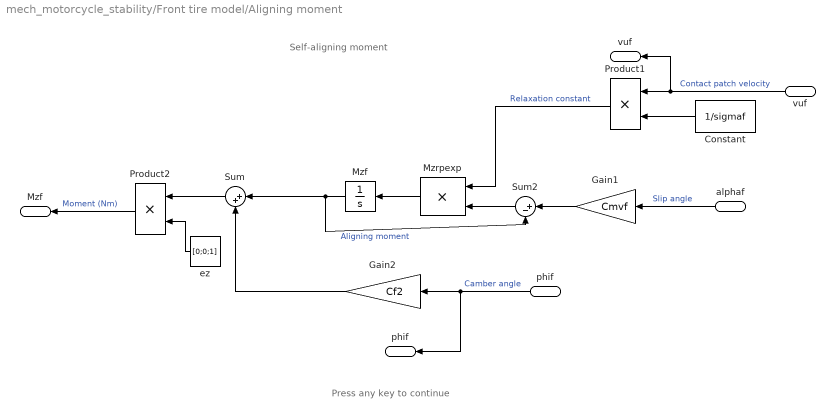
== system mech_motorcycle_stability/Front tire model/Aligning moment ==
  note: Self-aligning moment
  note: Press any key to continue
  vuf : Inport  Orientation=left  Port=1  LatchInput=off
  phif : Inport  Orientation=left  Port=2  LatchInput=off
  alphaf : Inport  Orientation=left  Port=3  LatchInput=off
  Constant : Constant  Orientation=left  Value=1/sigmaf
  Gain1 : Gain  Orientation=left  Gain=Cmvf  SaturateOnIntegerOverflow=on
  Gain2 : Gain  Orientation=left  Gain=Cf2  SaturateOnIntegerOverflow=on
  "Mzf  " : Integrator  Orientation=left  ZeroCross=off
  Mzrpexp : Product  Orientation=left  SaturateOnIntegerOverflow=on  InputSameDT=on
  Product1 : Product  Orientation=left  SaturateOnIntegerOverflow=on  InputSameDT=on
  Product2 : Product  Orientation=left  SaturateOnIntegerOverflow=on  InputSameDT=on
  Sum : Sum  Orientation=left  Inputs=|++  SaturateOnIntegerOverflow=on  InputSameDT=on
  Sum2 : Sum  Orientation=left  Inputs=|+-  SaturateOnIntegerOverflow=on  InputSameDT=on
  ez : Constant  Orientation=left  Value=[0;0;1]
  Mzf : Outport  Orientation=left
  "phif " : Outport  Orientation=left  Port=2
  "vuf " : Outport  Orientation=left  Port=3
  wires:
  Product2/1 -> Mzf/1  "Moment (Nm)"
  ez/1 -> Product2/2
  Sum/1 -> Product2/1
  Gain2/1 -> Sum/2
  phif/1 -> "phif "/1, Gain2/1  "Camber angle"
  alphaf/1 -> Gain1/1  "Slip angle"
  "Mzf  "/1 -> Sum2/2, Sum/1  "Aligning moment"
  Gain1/1 -> Sum2/1
  Sum2/1 -> Mzrpexp/2
  Product1/1 -> Mzrpexp/1  "Relaxation constant"
  Mzrpexp/1 -> "Mzf  "/1
  Constant/1 -> Product1/2
  vuf/1 -> Product1/1, "vuf "/1  "Contact patch velocity"

== system mech_motorcycle_stability/Front tire model/Contact ==
  note: Contact
  note: Press any key to continue
  Body Sensor : mblibv1/Sensors &  Actuators/Body Sensor  Orientation=left  Opaque=on  PhysicalDomain=Mechanical  PortType=blob  Muxed=off  Pose=on  Angle=on  AngleUnits=deg  ArcVelocity=off  ArcVelocityUnits=rad/s  ArcAcceleration=off  ArcAccelerationUnits=rad/s^2  CoordPosition=off  CoordPositionUnits=m  Velocity=on  VelocityUnits=m/s  Acceleration=off  AccelerationUnits=m/s^2  Quaternion=on  QuaternionDT=off  QuaternionDDT=off  QuaternionUnits=off  OutputVector=[ 3 9 ]  ActiveIO=on  Width=12  DialogClass=MechanicalSensorBlock  ReferenceFrame=Absolute (World)
  Contact geometry : Subsystem  Orientation=left
  Product1 : Product  Orientation=left  Multiplication=Matrix(*)  SaturateOnIntegerOverflow=on  InputSameDT=on
  Reshape : simulink/Math Operations/Reshape  Orientation=left  OutputDimensionality=Row vector  OutputDimensions=[1,1]
  Reshape1 : simulink/Math Operations/Reshape  Orientation=left  OutputDimensionality=Column vector  OutputDimensions=[1,1]
  Rear Wheel : PMIOPort  Orientation=left  Port=1  Side=Left
  fw_long : Outport  Orientation=left
  vuf : Outport  Orientation=left  Port=2
  phif : Outport  Orientation=left  Port=3
  dfwcp_dt : Outport  Orientation=left  Port=4
  fw_lat : Outport  Orientation=left  Port=5
  wires:
  Contact geometry/3(phif) -> phif/1  "Camber angle (rad)"
  Contact geometry/1(fw_lat) -> fw_lat/1  "Lateral direction"
  Body Sensor/2 -> Contact geometry/1(T)  "Body orientation"
  Reshape1/1 -> Product1/2
  Reshape/1 -> Product1/1
  Product1/1 -> vuf/1  "Longitudinal component (m/s)"
  Body Sensor/1 -> Reshape/1, dfwcp_dt/1  "Contact patch velocity (m/s)"
  Contact geometry/2(fw_long) -> fw_long/1, Reshape1/1  "Longitudinal direction"
  connections:
  Rear Wheel/RConn1 -- Body Sensor/LConn1

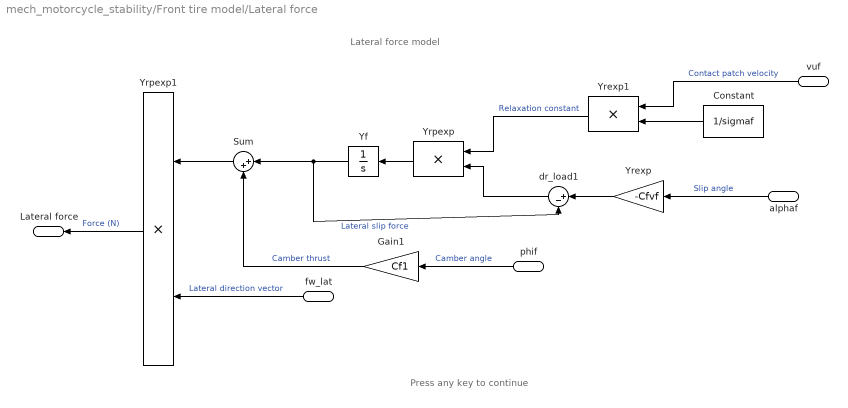
== system mech_motorcycle_stability/Front tire model/Lateral force ==
  note: Lateral force model
  note: Press any key to continue
  phif : Inport  Orientation=left  Port=1  LatchInput=off
  vuf : Inport  Orientation=left  Port=2  LatchInput=off
  alphaf : Inport  Orientation=left  Port=3  LatchInput=off
  fw_lat : Inport  Orientation=left  Port=4  LatchInput=off
  Constant : Constant  Orientation=left  Value=1/sigmaf
  Gain1 : Gain  Orientation=left  Gain=Cf1  SaturateOnIntegerOverflow=on
  Sum : Sum  Orientation=left  Inputs=|++  SaturateOnIntegerOverflow=on  InputSameDT=on
  Yf : Integrator  Orientation=left  ZeroCross=off
  Yrexp : Gain  Orientation=left  Gain=-Cfvf  SaturateOnIntegerOverflow=on
  Yrexp1 : Product  Orientation=left  SaturateOnIntegerOverflow=on  InputSameDT=on
  Yrpexp : Product  Orientation=left  SaturateOnIntegerOverflow=on  InputSameDT=on
  Yrpexp1 : Product  Orientation=left  SaturateOnIntegerOverflow=on  InputSameDT=on
  dr_load1 : Sum  Orientation=left  Inputs=|+-  SaturateOnIntegerOverflow=on  InputSameDT=on
  Lateral force : Outport  Orientation=left
  wires:
  Yrpexp1/1 -> Lateral force/1  "Force (N)"
  fw_lat/1 -> Yrpexp1/2  "Lateral direction vector"
  Sum/1 -> Yrpexp1/1
  Gain1/1 -> Sum/2  "Camber thrust"
  phif/1 -> Gain1/1  "Camber angle"
  alphaf/1 -> Yrexp/1  "Slip angle"
  Yrexp/1 -> dr_load1/1
  Yf/1 -> Sum/1, dr_load1/2  "Lateral slip force"
  Yrpexp/1 -> Yf/1
  dr_load1/1 -> Yrpexp/2
  Yrexp1/1 -> Yrpexp/1  "Relaxation constant"
  Constant/1 -> Yrexp1/2
  vuf/1 -> Yrexp1/1  "Contact patch velocity"

== system mech_motorcycle_stability/Front tire model/Lateral slip computation ==
  note: Lateral slip computation
  note: Press any key to continue
  dfwcp_dt : Inport  Orientation=left  Port=1  LatchInput=off
  fw_lat : Inport  Orientation=left  Port=2  LatchInput=off
  Fcn : Fcn  Orientation=left  Expr=1.0/sqrt(u[1]*u[1] + u[2]*u[2] + u[3]*u[3])
  Product : Product  Orientation=left  SaturateOnIntegerOverflow=on  InputSameDT=on
  Product1 : Product  Orientation=left  Multiplication=Matrix(*)  SaturateOnIntegerOverflow=on  InputSameDT=on
  Reshape : simulink/Math Operations/Reshape  Orientation=left  OutputDimensionality=Row vector  OutputDimensions=[1,1]
  Reshape1 : simulink/Math Operations/Reshape  Orientation=left  OutputDimensionality=Column vector  OutputDimensions=[1,1]
  Trigonometric Function : Trigonometry  Orientation=left  Operator=asin
  alphaf : Outport  Orientation=left
  wires:
  Product/1 -> Reshape/1  "Unit vector"
  Fcn/1 -> Product/1
  dfwcp_dt/1 -> Fcn/1, Product/2  "Velocity (m/s)"
  fw_lat/1 -> Reshape1/1  "Lateral direction"
  Reshape1/1 -> Product1/2
  Trigonometric Function/1 -> alphaf/1  "Slip angle (rad)"
  Product1/1 -> Trigonometric Function/1
  Reshape/1 -> Product1/1

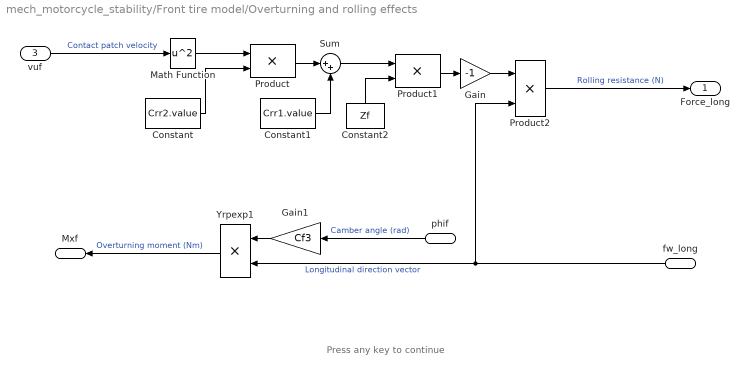
== system mech_motorcycle_stability/Front tire model/Overturning and rolling effects ==
  note: Press any key to continue
  fw_long : Inport  Orientation=left  Port=1  LatchInput=off
  phif : Inport  Orientation=left  Port=2  LatchInput=off
  vuf : Inport  Port=3  LatchInput=off
  Constant : Constant  Value=Crr2.value
  Constant1 : Constant  Value=Crr1.value
  Constant2 : Constant  Orientation=up  Value=Zf
  Gain : Gain  Gain=-1  SaturateOnIntegerOverflow=on
  Gain1 : Gain  Orientation=left  Gain=Cf3  SaturateOnIntegerOverflow=on
  Math Function : Math  Operator=square  SaturateOnIntegerOverflow=on
  Product : Product  SaturateOnIntegerOverflow=on  InputSameDT=on
  Product1 : Product  SaturateOnIntegerOverflow=on  InputSameDT=on
  Product2 : Product  SaturateOnIntegerOverflow=on  InputSameDT=on
  Sum : Sum  Inputs=|++  SaturateOnIntegerOverflow=on  InputSameDT=on
  Yrpexp1 : Product  Orientation=left  SaturateOnIntegerOverflow=on  InputSameDT=on
  Force_long : Outport
  Mxf : Outport  Orientation=left  Port=2
  wires:
  Yrpexp1/1 -> Mxf/1  "Overturning moment (Nm)"
  Gain1/1 -> Yrpexp1/1
  phif/1 -> Gain1/1  "Camber angle (rad)"
  Product2/1 -> Force_long/1  "Rolling resistance (N)"
  Gain/1 -> Product2/1
  Product1/1 -> Gain/1
  Constant2/1 -> Product1/2
  Sum/1 -> Product1/1
  Constant1/1 -> Sum/2
  Constant/1 -> Product/2
  Math Function/1 -> Product/1
  Product/1 -> Sum/1
  vuf/1 -> Math Function/1  "Contact patch velocity"
  fw_long/1 -> Yrpexp1/2, Product2/2  "Longitudinal direction vector"

== system mech_motorcycle_stability/Front tire model/Vertical force ==
  note: Press any key to continue
  Constant : Constant  Orientation=left  Value=-Zf
  Product2 : Product  Orientation=left  SaturateOnIntegerOverflow=on  InputSameDT=on
  ez : Constant  Orientation=left  Value=[0;0;1]
  Force_vert : Outport  Orientation=left
  wires:
  ez/1 -> Product2/2
  Constant/1 -> Product2/1
  Product2/1 -> Force_vert/1  "Vertical force (N)"

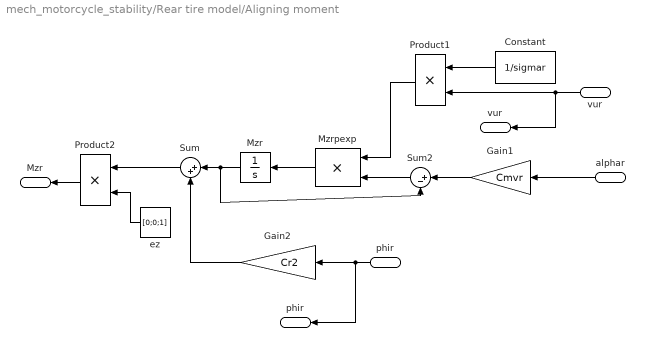
== system mech_motorcycle_stability/Rear tire model/Aligning moment ==
  vur : Inport  Orientation=left  Port=1  LatchInput=off
  phir : Inport  Orientation=left  Port=2  LatchInput=off
  alphar : Inport  Orientation=left  Port=3  LatchInput=off
  Constant : Constant  Orientation=left  Value=1/sigmar
  Gain1 : Gain  Orientation=left  Gain=Cmvr  SaturateOnIntegerOverflow=on
  Gain2 : Gain  Orientation=left  Gain=Cr2  SaturateOnIntegerOverflow=on
  "Mzr  " : Integrator  Orientation=left  ZeroCross=off
  Mzrpexp : Product  Orientation=left  SaturateOnIntegerOverflow=on  InputSameDT=on
  Product1 : Product  Orientation=left  SaturateOnIntegerOverflow=on  InputSameDT=on
  Product2 : Product  Orientation=left  SaturateOnIntegerOverflow=on  InputSameDT=on
  Sum : Sum  Orientation=left  Inputs=|++  SaturateOnIntegerOverflow=on  InputSameDT=on
  Sum2 : Sum  Orientation=left  Inputs=|+-  SaturateOnIntegerOverflow=on  InputSameDT=on
  ez : Constant  Orientation=left  Value=[0;0;1]
  Mzr : Outport  Orientation=left
  "phir " : Outport  Orientation=left  Port=2
  "vur " : Outport  Orientation=left  Port=3
  wires:
  Mzrpexp/1 -> "Mzr  "/1
  Product1/1 -> Mzrpexp/1
  Sum2/1 -> Mzrpexp/2
  vur/1 -> Product1/2, "vur "/1
  Gain1/1 -> Sum2/1
  "Mzr  "/1 -> Sum2/2, Sum/1
  alphar/1 -> Gain1/1
  Constant/1 -> Product1/1
  phir/1 -> Gain2/1, "phir "/1
  Gain2/1 -> Sum/2
  Sum/1 -> Product2/1
  ez/1 -> Product2/2
  Product2/1 -> Mzr/1

== system mech_motorcycle_stability/Rear tire model/Contact ==
  Body Sensor : mblibv1/Sensors &  Actuators/Body Sensor  Orientation=left  Opaque=on  PhysicalDomain=Mechanical  PortType=blob  Muxed=off  Pose=on  Angle=on  AngleUnits=deg  ArcVelocity=off  ArcVelocityUnits=rad/s  ArcAcceleration=off  ArcAccelerationUnits=rad/s^2  CoordPosition=off  CoordPositionUnits=m  Velocity=on  VelocityUnits=m/s  Acceleration=off  AccelerationUnits=m/s^2  Quaternion=on  QuaternionDT=off  QuaternionDDT=off  QuaternionUnits=off  OutputVector=[ 3 9 ]  ActiveIO=on  Width=12  DialogClass=MechanicalSensorBlock  ReferenceFrame=Absolute (World)
  Contact geometry : Subsystem  Orientation=left
  Product1 : Product  Orientation=left  Multiplication=Matrix(*)  SaturateOnIntegerOverflow=on  InputSameDT=on
  Reshape : simulink/Math Operations/Reshape  Orientation=left  OutputDimensionality=Row vector  OutputDimensions=[1,1]
  Reshape1 : simulink/Math Operations/Reshape  Orientation=left  OutputDimensionality=Column vector  OutputDimensions=[1,1]
  Rear Wheel : PMIOPort  Orientation=left  Port=1  Side=Left
  rw_long : Outport  Orientation=left
  vur : Outport  Orientation=left  Port=2
  phir : Outport  Orientation=left  Port=3
  drwcp_dt : Outport  Orientation=left  Port=4
  rw_lat : Outport  Orientation=left  Port=5
  wires:
  Body Sensor/2 -> Contact geometry/1(T)
  Contact geometry/1(rw_lat) -> rw_lat/1
  Contact geometry/3(phir) -> phir/1
  Reshape1/1 -> Product1/2
  Reshape/1 -> Product1/1
  Product1/1 -> vur/1
  Body Sensor/1 -> Reshape/1, drwcp_dt/1
  Contact geometry/2(rw_long) -> rw_long/1, Reshape1/1
  connections:
  Rear Wheel/RConn1 -- Body Sensor/LConn1
